simulink model "VehCtrl20260630_18B"  (R2018b)
settings: Solver=FixedStepAuto  StartTime=0.0  StopTime=inf  FixedStep=0.005  RelTol=1e-3
InitFcn:
  | mbd_mpc_consistency_checks(bdroot(gcs));
undefined symbols (not defined in the file): ANG_DEAD, BMS_NormalPwr, BrakeDeadZone, BrkPrsByBrkPct_TB_X, BrkPrsByBrkPct_TB_Y, DELAY_DISCHARGE, DELAY_RCUOFF, DRV_BACKWARD, DRV_BRAKE, DRV_FORWARD, DRV_NEUTRAL, DRV_PARK, DRV_UNPARK, DRV_ZEROTURN, EPB_LOCK, EPB_UNLOCK, ExtraLoadPwr, FanOff, fifo_0_vect, fifo_1_vect, HiFanReq, HV_finished, HV_No_Active, HV_POWER_OFF, HV_POWER_ON, HVDown, HVON, KaTLS_v_DrgUp_X_VehSpd, KeFTM_s_Way1OffDlyTime, KeFTM_TK_Way1CoolLv2OffBatTemp, KeFTM_TK_Way1CoolLv2OffMtrTemp, KeFTM_TK_Way1CoolLv2OnBatTemp, KeFTM_TK_Way1CoolLv2OnMtrTemp, KeFTM_TK_Way1CoolLv3OffBatTemp, KeFTM_TK_Way1CoolLv3OffMtrTemp, KeFTM_TK_Way1CoolLv3OnBatTemp, KeFTM_TK_Way1CoolLv3OnMtrTemp, KeFTM_TK_Way1CoolLv4OffBatTemp, KeFTM_TK_Way1CoolLv4OffMtrTemp, KeFTM_TK_Way1CoolLv4OnBatTemp, KeFTM_TK_Way1CoolLv4OnMtrTemp, Kp1, Kp2, LowFanReq, LQFP, MtrCmdGainFL, MtrCmdGainFR, MtrCmdGainRL, MtrCmdGainRR, MtrPwrFactor_RCU, MtrPwrHighToMidThd, MtrPwrLowToMidThd, MtrPwrMidToHighThd, MtrPwrMidToLowThd, MtrTrqMax, PCT_DEAD, Precharge, PTO_1000, PTO_540, pts1_fifo_0_vect ... (+32)
libraries: mbd_mpc574x_ec_toolbox x175, simulink x110, canmsglib x70
(part 2 of 15)

== system VehCtrl20260630_18B/Init ==
  CAN_init : Subsystem
  Data Store Read1 : DataStoreRead  DataStoreName=VCU_Mode
  Data Store Read3 : DataStoreRead  DataStoreName=Init_flg
  If1 : If  IfExpression=u1 == 2  ShowElse=off
  If2 : If  IfExpression=u1 == 0  ShowElse=off
  Init : Subsystem
  wires:
  Data Store Read3/1 -> If2/1
  If2/1 -> Init/Action
  Data Store Read1/1 -> If1/1
  If1/1 -> CAN_init/Action

== system VehCtrl20260630_18B/Initialization & SPI timer1 ==
  note: 由于SPI0用了两个片选，SPI3只用了一个片选（没算EEPROM）。
      | 因此直接用方波就可以了。
      | 如果增加SPI控制，建议使用StateFlow构造激活函数。
      | 由于模版使用的0.01s的仿真步长，这里构造周期为0.02s,占空比为0.5的方波。
  note: SPI3
  note: SPI0
  CS1 LS : Subsystem
  CS2 CANB : Subsystem
  CS3 LS : Subsystem
  CS5 LS : Subsystem
  Chart : Stateflow chart  TreatAsAtomicUnit=on
  Chart1 : Stateflow chart  TreatAsAtomicUnit=on
  Chart2 : Stateflow chart  TreatAsAtomicUnit=on
  Compare To Constant : simulink/Logic and Bit Operations/Compare To Constant  relop===  const=9  OutDataTypeStr=boolean
  Compare To Constant1 : simulink/Logic and Bit Operations/Compare To Constant  relop===  const=9  OutDataTypeStr=boolean
  Constant : Constant
  Data Store Read : DataStoreRead  DataStoreName=VCU_Mode
  Data Store Read1 : DataStoreRead  DataStoreName=ResetFlg
  Data Store Read2 : DataStoreRead  DataStoreName=Init_flg_SPI
  Data Store Write : DataStoreWrite  DataStoreName=VCU_Mode
  Data Store Write2 : DataStoreWrite  DataStoreName=SPI0_CS
  Data Store Write3 : DataStoreWrite  DataStoreName=SPI3_CS
  Data Store Write4 : DataStoreWrite  DataStoreName=Init_flg_SPI
  Data Type Conversion{,1..3} (4 alike) : DataTypeConversion
  If : If  IfExpression=u1 == 1  ShowElse=off
  If1 : If  IfExpression=u1 == 1  ShowElse=off
  If2 : If  IfExpression=u1 == 2  ShowElse=off
  If3 : If  IfExpression=u1 == 2  ShowElse=off
  Logical Operator : Logic  AllPortsSameDT=off  OutDataTypeStr=boolean
  Pulse Generator : DiscretePulseGenerator  PulseType=Time based  Period=0.01  PulseWidth=50
  wires:
  If/1 -> CS2 CANB/Action
  Chart/1(Flg) -> Data Type Conversion3/1
  Data Store Read2/1 -> Chart/2(InitFlg)
  If1/1 -> CS1 LS/Action
  Chart2/1(Flg) -> If3/1, [SPI3_flg], If/1
  Data Store Read/1 -> Chart2/1(VcuMode), Chart1/1(VcuMode)
  If2/1 -> CS5 LS/Action
  [SPI0_flg] -> Compare To Constant/1
  [SPI3_flg] -> Compare To Constant1/1
  Compare To Constant/1 -> Logical Operator/1
  Compare To Constant1/1 -> Logical Operator/2
  Logical Operator/1 -> Data Type Conversion2/1
  If3/1 -> CS3 LS/Action
  Pulse Generator/1 -> Data Type Conversion/1
  Constant/1 -> Data Type Conversion1/1
  Data Type Conversion/1 -> Data Store Write2/1
  Data Type Conversion1/1 -> Data Store Write3/1
  Data Type Conversion2/1 -> Data Store Write4/1
  Data Type Conversion3/1 -> Data Store Write/1
  Chart1/1(Flg) -> If1/1, [SPI0_flg], If2/1
  Data Store Read1/1 -> Chart/1(ResetFlg)

== system VehCtrl20260630_18B/Power Managment ==
  PowerMode : Inport
  Data Type Conversion : DataTypeConversion
  HS1 : mbd_mpc574x_ec_toolbox/GPIO Blocks/Digital_Output  Priority=1  gpio_pin=PTF6: [SIUL2_GPIO86 | General Purpose IO PF[6]]  gpio_drive_strength=Disabled
  HS4 : mbd_mpc574x_ec_toolbox/GPIO Blocks/Digital_Output  Priority=1  gpio_pin=PTA13: [SIUL2_GPIO13 | General Purpose IO PA[13]]  gpio_drive_strength=Disabled
  wires:
  PowerMode/1 -> Data Type Conversion/1
  Data Type Conversion/1 -> HS4/1, HS1/1

== system VehCtrl20260630_18B/SPI_EEPROM ==
  Data Store Memory : DataStoreMemory  DataStoreName=A_write  ReadBeforeWriteMsg=warning  WriteAfterWriteMsg=warning  WriteAfterReadMsg=warning  ShowAdditionalParam=off  OutDataTypeStr=single
      settings: RTWStateStorageClass=ExportedGlobal
  Data Store Memory10 : DataStoreMemory  DataStoreName=A_read  ReadBeforeWriteMsg=warning  WriteAfterWriteMsg=warning  WriteAfterReadMsg=warning  ShowAdditionalParam=off  OutDataTypeStr=single
      settings: RTWStateStorageClass=ExportedGlobal
  Data Store Memory18 : DataStoreMemory  DataStoreName=SPI0_CTRL0  ReadBeforeWriteMsg=warning  WriteAfterWriteMsg=warning  WriteAfterReadMsg=warning  ShowAdditionalParam=off  OutDataTypeStr=uint8
      settings: RTWStateStorageClass=ExportedGlobal
  Data Store Read : DataStoreRead  DataStoreName=SPI0_CTRL0
  SPI_read : Subsystem  TreatAsAtomicUnit=on
  SPI_write : Subsystem  TreatAsAtomicUnit=on
  Switch Case : SwitchCase  CaseConditions={1,2}  ShowDefaultCase=off
  wires:
  Data Store Read/1 -> Switch Case/1
  Switch Case/2 -> SPI_write/Action
  Switch Case/1 -> SPI_read/Action

== system VehCtrl20260630_18B/SigIn ==
  note: HardWareSignalIn
  note: CAN
  AI : Subsystem
  CAN0 : Subsystem  TreatAsAtomicUnit=on
      settings: RTWSystemCode=Nonreusable function
  CAN0_Rx_500 : mbd_mpc574x_ec_toolbox/Communication Blocks/CAN Blocks/FCAN_Isr  can_instance=0  can_event=Rx Complete
      settings: SourceProductName=NXP Model-Based Design Toolbox for MPC57xx MCUs
  CAN1 : Subsystem  TreatAsAtomicUnit=on
      settings: RTWSystemCode=Nonreusable function
  CAN1_Rx_500 : mbd_mpc574x_ec_toolbox/Communication Blocks/CAN Blocks/FCAN_Isr  can_instance=1  can_event=Rx Complete
      settings: SourceProductName=NXP Model-Based Design Toolbox for MPC57xx MCUs
  DI : Subsystem
  PWM : Subsystem
  Terminator{,3..5,8} (5 alike) : Terminator
  MCU_FL : Outport  VectorParamsAs1DForOutWhenUnconnected=on
  MCU_FR : Outport  Port=2  VectorParamsAs1DForOutWhenUnconnected=on
  MCU_RL : Outport  Port=3  VectorParamsAs1DForOutWhenUnconnected=on
  MCU_RR : Outport  Port=4  VectorParamsAs1DForOutWhenUnconnected=on
  MCU_PTO : Outport  Port=5  VectorParamsAs1DForOutWhenUnconnected=on
  BMS : Outport  Port=6  VectorParamsAs1DForOutWhenUnconnected=on
  DCDC : Outport  Port=7  VectorParamsAs1DForOutWhenUnconnected=on
  BDX : Outport  Port=8  VectorParamsAs1DForOutWhenUnconnected=on
  ACM : Outport  Port=9  VectorParamsAs1DForOutWhenUnconnected=on
  RCU : Outport  Port=10  VectorParamsAs1DForOutWhenUnconnected=on
  RMT : Outport  Port=11  VectorParamsAs1DForOutWhenUnconnected=on
  PTC : Outport  Port=12
  AUTO : Outport  Port=13  VectorParamsAs1DForOutWhenUnconnected=on
  wires:
  CAN0_Rx_500/2 -> Terminator4/1
  CAN0_Rx_500/6 -> CAN0/4(timestamp)
  CAN0_Rx_500/4 -> CAN0/2(Data)
  CAN0_Rx_500/3 -> CAN0/1(ID)
  CAN0_Rx_500/5 -> CAN0/3(length)
  CAN1_Rx_500/5 -> CAN1/3(length)
  CAN1_Rx_500/3 -> CAN1/1(ID)
  CAN1_Rx_500/4 -> CAN1/2(Data)
  CAN1_Rx_500/6 -> CAN1/4(timestamp)
  CAN1_Rx_500/1 -> CAN1/Trigger
  CAN1_Rx_500/2 -> Terminator8/1
  CAN1/1(MCU_FL) -> MCU_FL/1
  CAN1/2(MCU_FR) -> MCU_FR/1
  CAN1/4(MCU_RR) -> MCU_RR/1
  CAN1/3(MCU_RL) -> MCU_RL/1
  CAN0_Rx_500/1 -> CAN0/Trigger
  CAN1/5(MCU_PTO) -> MCU_PTO/1
  CAN1/6(BMS) -> BMS/1
  CAN1/7(BDX) -> BDX/1
  CAN0/3(DCDC) -> DCDC/1
  CAN1/8(ACM) -> ACM/1
  CAN1/9(RCU) -> RCU/1
  CAN0/1(PTC) -> PTC/1
  CAN0/4(RMT) -> RMT/1
  PWM/1(PWMIn) -> Terminator/1
  DI/1(DI) -> Terminator3/1
  AI/1(AI) -> Terminator5/1
  CAN0/2(AUTO) -> AUTO/1

== system VehCtrl20260630_18B/SigOut ==
  BMS_OUT : Inport
  RCU_OUT : Inport  Port=2
  DCDC_OUT : Inport  Port=3
  MCU_OUT : Inport  Port=4
  BDX_OUT : Inport  Port=5
  CAN_INFO : Inport  Port=6
  AUTO : Subsystem
  BDX : Subsystem  TreatAsAtomicUnit=on  SystemSampleTime=0.01
  BMS : Subsystem  TreatAsAtomicUnit=on  SystemSampleTime=0.01
  DCDC : Subsystem  TreatAsAtomicUnit=on  SystemSampleTime=0.01
  "GPIO " : Subsystem
  MCU : Subsystem  TreatAsAtomicUnit=on  SystemSampleTime=0.01
  METER : Subsystem
  PTC_ACM : Subsystem  TreatAsAtomicUnit=on  SystemSampleTime=0.01
  Pulse Generator : DiscretePulseGenerator  PulseType=Time based  Period=0.1  PulseWidth=5
  Pulse Generator1 : DiscretePulseGenerator  PulseType=Time based  Period=0.01  PulseWidth=50
  Pulse Generator2 : DiscretePulseGenerator  PulseType=Time based  Period=0.02  PulseWidth=25
  Pulse Generator3 : DiscretePulseGenerator  PulseType=Time based  Period=0.1  PulseWidth=5
  Pulse Generator4 : DiscretePulseGenerator  PulseType=Time based  Period=0.01  PulseWidth=50
  Pulse Generator5 : DiscretePulseGenerator  PulseType=Time based  Period=0.2  PulseWidth=50
  RCU : Subsystem  TreatAsAtomicUnit=on  SystemSampleTime=0.01
  Rate Transition{,1..5} (6 alike) : RateTransition
  wires:
  Rate Transition5/1 -> METER/1("CAN_INFO "), AUTO/1("CAN_INFO ")
  Pulse Generator2/1 -> BDX/Trigger
  Pulse Generator5/1 -> METER/Trigger
  BMS_OUT/1 -> Rate Transition/1
  Pulse Generator1/1 -> MCU/Trigger, RCU/Trigger
  MCU_OUT/1 -> Rate Transition3/1
  Pulse Generator3/1 -> PTC_ACM/Trigger
  Rate Transition2/1 -> DCDC/1("DCDC_OUT ")
  Rate Transition/1 -> BMS/1("BMS_OUT ")
  Rate Transition4/1 -> BDX/1("BDX_OUT ")
  RCU_OUT/1 -> Rate Transition1/1
  CAN_INFO/1 -> Rate Transition5/1
  Pulse Generator4/1 -> AUTO/Trigger
  Rate Transition1/1 -> RCU/1("RCU_OUT ")
  DCDC_OUT/1 -> Rate Transition2/1
  Pulse Generator/1 -> DCDC/Trigger, BMS/Trigger
  BDX_OUT/1 -> Rate Transition4/1
  Rate Transition3/1 -> MCU/1("MCU_OUT_FL ")

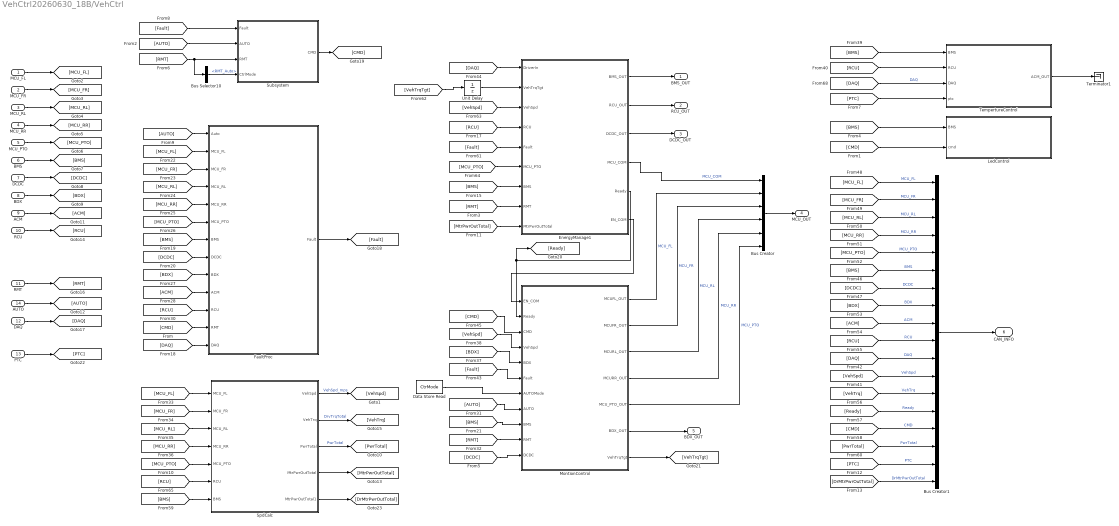
== system VehCtrl20260630_18B/VehCtrl ==
  MCU_FL : Inport
  MCU_FR : Inport  Port=2
  MCU_RL : Inport  Port=3
  MCU_RR : Inport  Port=4
  MCU_PTO : Inport  Port=5
  BMS : Inport  Port=6
  DCDC : Inport  Port=7
  BDX : Inport  Port=8
  ACM : Inport  Port=9
  RCU : Inport  Port=10
  RMT : Inport  Port=11
  DAQ : Inport  Port=12
  "PTC " : Inport  Port=13
  AUTO : Inport  Port=14
  Bus Creator : BusCreator  Inputs=6
  Bus Creator1 : BusCreator  Inputs=18
  Bus Selector10 : BusSelector  OutputSignals=RMT3.RMT_Auto
  Data Store Read : DataStoreRead  DataStoreName=CtrMode
  EnergyManage1 : Subsystem
  FaultProc : Subsystem
  LedControl : Subsystem
  MontionControl : Subsystem
  SpdCalc : Subsystem
  Subsystem : Subsystem
  TempertureControl : Subsystem
  Terminator1 : Terminator
  Unit Delay : UnitDelay  SampleTime=-1
  BMS_OUT : Outport
  RCU_OUT : Outport  Port=2
  DCDC_OUT : Outport  Port=3
  MCU_OUT : Outport  Port=4
  BDX_OUT : Outport  Port=5
  CAN_INFO : Outport  Port=6
  wires:
  MCU_FL/1 -> [MCU_FL]
  MCU_FR/1 -> [MCU_FR]
  MCU_RR/1 -> [MCU_RR]
  MCU_RL/1 -> [MCU_RL]
  DCDC/1 -> [DCDC]
  BDX/1 -> [BDX]
  BMS/1 -> [BMS]
  MCU_PTO/1 -> [MCU_PTO]
  RMT/1 -> [RMT]
  DAQ/1 -> [DAQ]
  RCU/1 -> [RCU]
  ACM/1 -> [ACM]
  [RCU] -> EnergyManage1/4(RCU)
  [MCU_FL] -> FaultProc/2(MCU_FL)
  [MCU_FR] -> FaultProc/3(MCU_FR)
  [MCU_RL] -> FaultProc/4(MCU_RL)
  [MCU_RR] -> FaultProc/5(MCU_RR)
  [MCU_PTO] -> FaultProc/6(MCU_PTO)
  [BMS] -> FaultProc/7(BMS)
  [DCDC] -> FaultProc/8(DCDC)
  [BDX] -> FaultProc/9(BDX)
  [ACM] -> FaultProc/10(ACM)
  [RCU] -> FaultProc/11(RCU)
  [CMD] -> FaultProc/12(RMT)
  [DAQ] -> FaultProc/13(DAQ)
  [BDX] -> MontionControl/5(BDX)
  [VehSpd] -> MontionControl/4(VehSpd)
  FaultProc/1(Fault) -> [Fault]
  [Fault] -> MontionControl/6(Fault)
  [DAQ] -> EnergyManage1/1(DriverIn)
  [CMD] -> MontionControl/3(CMD)
  [Fault] -> EnergyManage1/5(Fault)
  MontionControl/7(VehTrqTgt) -> [VehTrqTgt]
  [VehTrqTgt] -> Unit Delay/1
  [VehSpd] -> EnergyManage1/3(VehSpd)
  [MCU_PTO] -> EnergyManage1/6(MCU_PTO)
  [BMS] -> EnergyManage1/7(BMS)
  Unit Delay/1 -> EnergyManage1/2(VehTrqTgt)
  EnergyManage1/4(MCU_COM) -> Bus Creator/1  "MCU_COM"
  Bus Creator/1 -> MCU_OUT/1
  EnergyManage1/1(BMS_OUT) -> BMS_OUT/1
  EnergyManage1/2(RCU_OUT) -> RCU_OUT/1
  EnergyManage1/3(DCDC_OUT) -> DCDC_OUT/1
  MontionControl/1(MCUFL_OUT) -> Bus Creator/2  "MCU_FL"
  MontionControl/2(MCUFR_OUT) -> Bus Creator/3  "MCU_FR"
  MontionControl/3(MCURL_OUT) -> Bus Creator/4  "MCU_RL"
  MontionControl/4(MCURR_OUT) -> Bus Creator/5  "MCU_RR"
  MontionControl/5(MCU_PTO_OUT) -> Bus Creator/6  "MCU_PTO"
  MontionControl/6(BDX_OUT) -> BDX_OUT/1
  "PTC "/1 -> [PTC]
  AUTO/1 -> [AUTO]
  [AUTO] -> Subsystem/2(AUTO)
  Subsystem/1(CMD) -> [CMD]
  Data Store Read/1 -> MontionControl/7(AUTOMode)
  [AUTO] -> MontionControl/8(AUTO)
  Bus Selector10/1 -> Subsystem/4(CtrlMode)  "<RMT_Auto>"
  [RMT] -> Subsystem/3(RMT), Bus Selector10/1
  [RMT] -> EnergyManage1/8("RMT ")
  [CMD] -> LedControl/2(cmd)
  TempertureControl/1(ACM_OUT) -> Terminator1/1
  [RCU] -> TempertureControl/2(RCU)
  [BMS] -> TempertureControl/1(BMS)
  [BMS] -> MontionControl/9(BMS)
  [RMT] -> MontionControl/10(RMT)
  [DAQ] -> TempertureControl/3(DAQ)  "DAQ"
  [BMS] -> LedControl/1(BMS)
  [DCDC] -> MontionControl/11(DCDC)
  [PTC] -> TempertureControl/4(ptc)
  [Fault] -> Subsystem/1(Fault)
  [AUTO] -> FaultProc/1(Auto)
  [MCU_RR] -> SpdCalc/4(MCU_RR)
  [MCU_FR] -> SpdCalc/2(MCU_FR)
  [MCU_FL] -> SpdCalc/1(MCU_FL)
  [MCU_PTO] -> SpdCalc/5(MCU_PTO)
  [BMS] -> SpdCalc/7(BMS)
  SpdCalc/2("VehTrq ") -> [VehTrq]  "DrvTrqTotal"
  [RCU] -> SpdCalc/6(RCU)
  SpdCalc/5(MtrPwrOutTotal1) -> [DrMtrPwrOutTotal]
  SpdCalc/4(MtrPwrOutTotal) -> [MtrPwrOutTotal]
  SpdCalc/1(VehSpd) -> [VehSpd]  "VehSpd_mps"
  SpdCalc/3(PwrTotal) -> [PwrTotal]  "PwrTotal"
  [MCU_RL] -> SpdCalc/3(MCU_RL)
  EnergyManage1/6(EN_COM) -> MontionControl/1(EN_COM)
  EnergyManage1/5(Ready) -> MontionControl/2(Ready), [Ready]
  [MtrPwrOutTotal] -> EnergyManage1/9(MtrPwrOutTotal)
  Bus Creator1/1 -> CAN_INFO/1
  [BMS] -> Bus Creator1/6  "BMS"
  [MCU_FR] -> Bus Creator1/2  "MCU_FR"
  [PwrTotal] -> Bus Creator1/16  "PwrTotal"
  [MCU_RL] -> Bus Creator1/3  "MCU_RL"
  [DAQ] -> Bus Creator1/11  "DAQ"
  [BDX] -> Bus Creator1/8  "BDX"
  [MCU_RR] -> Bus Creator1/4  "MCU_RR"
  [VehSpd] -> Bus Creator1/12  "VehSpd"
  [CMD] -> Bus Creator1/15  "CMD"
  [DrMtrPwrOutTotal] -> Bus Creator1/18  "DrMtrPwrOutTotal"
  [ACM] -> Bus Creator1/9  "ACM"
  [Ready] -> Bus Creator1/14  "Ready"
  [MCU_PTO] -> Bus Creator1/5  "MCU_PTO"
  [PTC] -> Bus Creator1/17  "PTC"
  [DCDC] -> Bus Creator1/7  "DCDC"
  [MCU_FL] -> Bus Creator1/1  "MCU_FL"
  [VehTrq] -> Bus Creator1/13  "VehTrq"
  [RCU] -> Bus Creator1/10  "RCU"

== system VehCtrl20260630_18B/Init/CAN_init ==
  note: CAN1
  note: CAN2
  Action Port : ActionPort  ActionType=then
  ACM : mbd_mpc574x_ec_toolbox/Communication Blocks/CAN Blocks/FCAN_Receive  can_instance=2  can_mode=Non-blocking  can_timeout_ms=0  can_mb_idx=28  can_extended_id=off  can_is_remote=off  can_id=284  can_msg_mask=FFFFFFFF  show_adv_opts=off  can_use_rxfifo=off  can_fd_enable=off
      settings: SourceProductName=NXP Model-Based Design Toolbox for MPC57xx MCUs
  AUTO1 : mbd_mpc574x_ec_toolbox/Communication Blocks/CAN Blocks/FCAN_Receive  can_instance=1  can_mode=Non-blocking  can_timeout_ms=0  can_mb_idx=37  can_extended_id=on  can_is_remote=off  can_id=1001  can_msg_mask=FFFFFFFF  show_adv_opts=off  can_use_rxfifo=off  can_fd_enable=off
      settings: SourceProductName=NXP Model-Based Design Toolbox for MPC57xx MCUs
  AUTO2 : mbd_mpc574x_ec_toolbox/Communication Blocks/CAN Blocks/FCAN_Receive  can_instance=1  can_mode=Non-blocking  can_timeout_ms=0  can_mb_idx=38  can_extended_id=on  can_is_remote=off  can_id=1002  can_msg_mask=FFFFFFFF  show_adv_opts=off  can_use_rxfifo=off  can_fd_enable=off
      settings: SourceProductName=NXP Model-Based Design Toolbox for MPC57xx MCUs
  AUTO3 : mbd_mpc574x_ec_toolbox/Communication Blocks/CAN Blocks/FCAN_Receive  can_instance=1  can_mode=Non-blocking  can_timeout_ms=0  can_mb_idx=61  can_extended_id=on  can_is_remote=off  can_id=1003  can_msg_mask=FFFFFFFF  show_adv_opts=off  can_use_rxfifo=off  can_fd_enable=off
      settings: SourceProductName=NXP Model-Based Design Toolbox for MPC57xx MCUs
  "BDX " : mbd_mpc574x_ec_toolbox/Communication Blocks/CAN Blocks/FCAN_Receive  can_instance=2  can_mode=Non-blocking  can_timeout_ms=0  can_mb_idx=27  can_extended_id=off  can_is_remote=off  can_id=180  can_msg_mask=FFFFFFFF  show_adv_opts=off  can_use_rxfifo=off  can_fd_enable=off
      settings: SourceProductName=NXP Model-Based Design Toolbox for MPC57xx MCUs
  BMS1 : mbd_mpc574x_ec_toolbox/Communication Blocks/CAN Blocks/FCAN_Receive  can_instance=2  can_mode=Non-blocking  can_timeout_ms=0  can_mb_idx=20  can_extended_id=on  can_is_remote=off  can_id=18012947  can_msg_mask=FFFFFFFF  show_adv_opts=off  can_use_rxfifo=off  can_fd_enable=off
      settings: SourceProductName=NXP Model-Based Design Toolbox for MPC57xx MCUs
  BMS10 : mbd_mpc574x_ec_toolbox/Communication Blocks/CAN Blocks/FCAN_Receive  can_instance=2  can_mode=Non-blocking  can_timeout_ms=0  can_mb_idx=54  can_extended_id=on  can_is_remote=off  can_id=18022947  can_msg_mask=FFFFFFFF  show_adv_opts=off  can_use_rxfifo=off  can_fd_enable=off
      settings: SourceProductName=NXP Model-Based Design Toolbox for MPC57xx MCUs
  BMS11 : mbd_mpc574x_ec_toolbox/Communication Blocks/CAN Blocks/FCAN_Receive  can_instance=2  can_mode=Non-blocking  can_timeout_ms=0  can_mb_idx=55  can_extended_id=on  can_is_remote=off  can_id=18032947  can_msg_mask=FFFFFFFF  show_adv_opts=off  can_use_rxfifo=off  can_fd_enable=off
      settings: SourceProductName=NXP Model-Based Design Toolbox for MPC57xx MCUs
  BMS12 : mbd_mpc574x_ec_toolbox/Communication Blocks/CAN Blocks/FCAN_Receive  Commented=on  can_instance=2  can_mode=Non-blocking  can_timeout_ms=0  can_mb_idx=56  can_extended_id=on  can_is_remote=off  can_id=1C1F7547  can_msg_mask=FFFFFFFF  show_adv_opts=off  can_use_rxfifo=off  can_fd_enable=off
      settings: SourceProductName=NXP Model-Based Design Toolbox for MPC57xx MCUs
  BMS2 : mbd_mpc574x_ec_toolbox/Communication Blocks/CAN Blocks/FCAN_Receive  can_instance=2  can_mode=Non-blocking  can_timeout_ms=0  can_mb_idx=21  can_extended_id=on  can_is_remote=off  can_id=18042947  can_msg_mask=FFFFFFFF  show_adv_opts=off  can_use_rxfifo=off  can_fd_enable=off
      settings: SourceProductName=NXP Model-Based Design Toolbox for MPC57xx MCUs
  BMS3 : mbd_mpc574x_ec_toolbox/Communication Blocks/CAN Blocks/FCAN_Receive  can_instance=2  can_mode=Non-blocking  can_timeout_ms=0  can_mb_idx=22  can_extended_id=on  can_is_remote=off  can_id=18052947  can_msg_mask=FFFFFFFF  show_adv_opts=off  can_use_rxfifo=off  can_fd_enable=off
      settings: SourceProductName=NXP Model-Based Design Toolbox for MPC57xx MCUs
  BMS4 : mbd_mpc574x_ec_toolbox/Communication Blocks/CAN Blocks/FCAN_Receive  Commented=on  can_instance=2  can_mode=Non-blocking  can_timeout_ms=0  can_mb_idx=23  can_extended_id=on  can_is_remote=off  can_id=18062947  can_msg_mask=FFFFFFFF  show_adv_opts=off  can_use_rxfifo=off  can_fd_enable=off
      settings: SourceProductName=NXP Model-Based Design Toolbox for MPC57xx MCUs
  BMS5 : mbd_mpc574x_ec_toolbox/Communication Blocks/CAN Blocks/FCAN_Receive  can_instance=2  can_mode=Non-blocking  can_timeout_ms=0  can_mb_idx=24  can_extended_id=on  can_is_remote=off  can_id=1C017547  can_msg_mask=FFFFFFFF  show_adv_opts=off  can_use_rxfifo=off  can_fd_enable=off
      settings: SourceProductName=NXP Model-Based Design Toolbox for MPC57xx MCUs
  BMS6 : mbd_mpc574x_ec_toolbox/Communication Blocks/CAN Blocks/FCAN_Receive  can_instance=2  can_mode=Non-blocking  can_timeout_ms=0  can_mb_idx=50  can_extended_id=on  can_is_remote=off  can_id=1C067547  can_msg_mask=FFFFFFFF  show_adv_opts=off  can_use_rxfifo=off  can_fd_enable=off
      settings: SourceProductName=NXP Model-Based Design Toolbox for MPC57xx MCUs
  BMS7 : mbd_mpc574x_ec_toolbox/Communication Blocks/CAN Blocks/FCAN_Receive  Commented=on  can_instance=2  can_mode=Non-blocking  can_timeout_ms=0  can_mb_idx=51  can_extended_id=on  can_is_remote=off  can_id=180D2947  can_msg_mask=FFFFFFFF  show_adv_opts=off  can_use_rxfifo=off  can_fd_enable=off
      settings: SourceProductName=NXP Model-Based Design Toolbox for MPC57xx MCUs
  BMS8 : mbd_mpc574x_ec_toolbox/Communication Blocks/CAN Blocks/FCAN_Receive  can_instance=2  can_mode=Non-blocking  can_timeout_ms=0  can_mb_idx=52  can_extended_id=on  can_is_remote=off  can_id=18602947  can_msg_mask=FFFFFFFF  show_adv_opts=off  can_use_rxfifo=off  can_fd_enable=off
      settings: SourceProductName=NXP Model-Based Design Toolbox for MPC57xx MCUs
  BMS9 : mbd_mpc574x_ec_toolbox/Communication Blocks/CAN Blocks/FCAN_Receive  can_instance=2  can_mode=Non-blocking  can_timeout_ms=0  can_mb_idx=53  can_extended_id=on  can_is_remote=off  can_id=18202947  can_msg_mask=FFFFFFFF  show_adv_opts=off  can_use_rxfifo=off  can_fd_enable=off
      settings: SourceProductName=NXP Model-Based Design Toolbox for MPC57xx MCUs
  DCDC : mbd_mpc574x_ec_toolbox/Communication Blocks/CAN Blocks/FCAN_Receive  can_instance=1  can_mode=Non-blocking  can_timeout_ms=0  can_mb_idx=26  can_extended_id=on  can_is_remote=off  can_id=18F8622B  can_msg_mask=FFFFFFFF  show_adv_opts=off  can_use_rxfifo=off  can_fd_enable=off
      settings: SourceProductName=NXP Model-Based Design Toolbox for MPC57xx MCUs
  MCU_FL1 : mbd_mpc574x_ec_toolbox/Communication Blocks/CAN Blocks/FCAN_Receive  can_instance=2  can_mode=Non-blocking  can_timeout_ms=0  can_mb_idx=12  can_extended_id=on  can_is_remote=off  can_id=C08A7F3  can_msg_mask=FFFFFFFF  show_adv_opts=off  can_use_rxfifo=off  can_fd_enable=off
      settings: SourceProductName=NXP Model-Based Design Toolbox for MPC57xx MCUs
  MCU_FL2 : mbd_mpc574x_ec_toolbox/Communication Blocks/CAN Blocks/FCAN_Receive  can_instance=2  can_mode=Non-blocking  can_timeout_ms=0  can_mb_idx=13  can_extended_id=on  can_is_remote=off  can_id=C09A7F3  can_msg_mask=FFFFFFFF  show_adv_opts=off  can_use_rxfifo=off  can_fd_enable=off
      settings: SourceProductName=NXP Model-Based Design Toolbox for MPC57xx MCUs
  MCU_FL3 : mbd_mpc574x_ec_toolbox/Communication Blocks/CAN Blocks/FCAN_Receive  can_instance=2  can_mode=Non-blocking  can_timeout_ms=0  can_mb_idx=14  can_extended_id=on  can_is_remote=off  can_id=C0AA7F3  can_msg_mask=FFFFFFFF  show_adv_opts=off  can_use_rxfifo=off  can_fd_enable=off
      settings: SourceProductName=NXP Model-Based Design Toolbox for MPC57xx MCUs
  MCU_FL4 : mbd_mpc574x_ec_toolbox/Communication Blocks/CAN Blocks/FCAN_Receive  Commented=on  can_instance=2  can_mode=Non-blocking  can_timeout_ms=0  can_mb_idx=15  can_extended_id=on  can_is_remote=off  can_id=C0BA7F3  can_msg_mask=FFFFFFFF  show_adv_opts=off  can_use_rxfifo=off  can_fd_enable=off
      settings: SourceProductName=NXP Model-Based Design Toolbox for MPC57xx MCUs
  MCU_FR1 : mbd_mpc574x_ec_toolbox/Communication Blocks/CAN Blocks/FCAN_Receive  can_instance=2  can_mode=Non-blocking  can_timeout_ms=0  can_mb_idx=0  can_extended_id=on  can_is_remote=off  can_id=C08A7F0  can_msg_mask=FFFFFFFF  show_adv_opts=off  can_use_rxfifo=off  can_fd_enable=off
      settings: SourceProductName=NXP Model-Based Design Toolbox for MPC57xx MCUs
  MCU_FR2 : mbd_mpc574x_ec_toolbox/Communication Blocks/CAN Blocks/FCAN_Receive  can_instance=2  can_mode=Non-blocking  can_timeout_ms=0  can_mb_idx=1  can_extended_id=on  can_is_remote=off  can_id=C09A7F0  can_msg_mask=FFFFFFFF  show_adv_opts=off  can_use_rxfifo=off  can_fd_enable=off
      settings: SourceProductName=NXP Model-Based Design Toolbox for MPC57xx MCUs
  MCU_FR3 : mbd_mpc574x_ec_toolbox/Communication Blocks/CAN Blocks/FCAN_Receive  can_instance=2  can_mode=Non-blocking  can_timeout_ms=0  can_mb_idx=2  can_extended_id=on  can_is_remote=off  can_id=C0AA7F0  can_msg_mask=FFFFFFFF  show_adv_opts=off  can_use_rxfifo=off  can_fd_enable=off
      settings: SourceProductName=NXP Model-Based Design Toolbox for MPC57xx MCUs
  MCU_FR4 : mbd_mpc574x_ec_toolbox/Communication Blocks/CAN Blocks/FCAN_Receive  Commented=on  can_instance=2  can_mode=Non-blocking  can_timeout_ms=0  can_mb_idx=3  can_extended_id=on  can_is_remote=off  can_id=C0BA7F0  can_msg_mask=FFFFFFFF  show_adv_opts=off  can_use_rxfifo=off  can_fd_enable=off
      settings: SourceProductName=NXP Model-Based Design Toolbox for MPC57xx MCUs
  MCU_PTO1 : mbd_mpc574x_ec_toolbox/Communication Blocks/CAN Blocks/FCAN_Receive  can_instance=2  can_mode=Non-blocking  can_timeout_ms=0  can_mb_idx=16  can_extended_id=on  can_is_remote=off  can_id=C08A7F4  can_msg_mask=FFFFFFFF  show_adv_opts=off  can_use_rxfifo=off  can_fd_enable=off
      settings: SourceProductName=NXP Model-Based Design Toolbox for MPC57xx MCUs
  MCU_PTO2 : mbd_mpc574x_ec_toolbox/Communication Blocks/CAN Blocks/FCAN_Receive  can_instance=2  can_mode=Non-blocking  can_timeout_ms=0  can_mb_idx=17  can_extended_id=on  can_is_remote=off  can_id=C09A7F4  can_msg_mask=FFFFFFFF  show_adv_opts=off  can_use_rxfifo=off  can_fd_enable=off
      settings: SourceProductName=NXP Model-Based Design Toolbox for MPC57xx MCUs
  MCU_PTO3 : mbd_mpc574x_ec_toolbox/Communication Blocks/CAN Blocks/FCAN_Receive  can_instance=2  can_mode=Non-blocking  can_timeout_ms=0  can_mb_idx=18  can_extended_id=on  can_is_remote=off  can_id=C0AA7F4  can_msg_mask=FFFFFFFF  show_adv_opts=off  can_use_rxfifo=off  can_fd_enable=off
      settings: SourceProductName=NXP Model-Based Design Toolbox for MPC57xx MCUs
  MCU_PTO4 : mbd_mpc574x_ec_toolbox/Communication Blocks/CAN Blocks/FCAN_Receive  Commented=on  can_instance=2  can_mode=Non-blocking  can_timeout_ms=0  can_mb_idx=19  can_extended_id=on  can_is_remote=off  can_id=C0BA7F4  can_msg_mask=FFFFFFFF  show_adv_opts=off  can_use_rxfifo=off  can_fd_enable=off
      settings: SourceProductName=NXP Model-Based Design Toolbox for MPC57xx MCUs
  MCU_RL1 : mbd_mpc574x_ec_toolbox/Communication Blocks/CAN Blocks/FCAN_Receive  can_instance=2  can_mode=Non-blocking  can_timeout_ms=0  can_mb_idx=8  can_extended_id=on  can_is_remote=off  can_id=C08A7F2  can_msg_mask=FFFFFFFF  show_adv_opts=off  can_use_rxfifo=off  can_fd_enable=off
      settings: SourceProductName=NXP Model-Based Design Toolbox for MPC57xx MCUs
  MCU_RL2 : mbd_mpc574x_ec_toolbox/Communication Blocks/CAN Blocks/FCAN_Receive  can_instance=2  can_mode=Non-blocking  can_timeout_ms=0  can_mb_idx=9  can_extended_id=on  can_is_remote=off  can_id=C09A7F2  can_msg_mask=FFFFFFFF  show_adv_opts=off  can_use_rxfifo=off  can_fd_enable=off
      settings: SourceProductName=NXP Model-Based Design Toolbox for MPC57xx MCUs
  MCU_RL3 : mbd_mpc574x_ec_toolbox/Communication Blocks/CAN Blocks/FCAN_Receive  can_instance=2  can_mode=Non-blocking  can_timeout_ms=0  can_mb_idx=10  can_extended_id=on  can_is_remote=off  can_id=C0AA7F2  can_msg_mask=FFFFFFFF  show_adv_opts=off  can_use_rxfifo=off  can_fd_enable=off
      settings: SourceProductName=NXP Model-Based Design Toolbox for MPC57xx MCUs
  MCU_RL4 : mbd_mpc574x_ec_toolbox/Communication Blocks/CAN Blocks/FCAN_Receive  Commented=on  can_instance=2  can_mode=Non-blocking  can_timeout_ms=0  can_mb_idx=11  can_extended_id=on  can_is_remote=off  can_id=C0BA7F2  can_msg_mask=FFFFFFFF  show_adv_opts=off  can_use_rxfifo=off  can_fd_enable=off
      settings: SourceProductName=NXP Model-Based Design Toolbox for MPC57xx MCUs
  MCU_RR1 : mbd_mpc574x_ec_toolbox/Communication Blocks/CAN Blocks/FCAN_Receive  can_instance=2  can_mode=Non-blocking  can_timeout_ms=0  can_mb_idx=4  can_extended_id=on  can_is_remote=off  can_id=C08A7F1  can_msg_mask=FFFFFFFF  show_adv_opts=off  can_use_rxfifo=off  can_fd_enable=off
      settings: SourceProductName=NXP Model-Based Design Toolbox for MPC57xx MCUs
  MCU_RR2 : mbd_mpc574x_ec_toolbox/Communication Blocks/CAN Blocks/FCAN_Receive  can_instance=2  can_mode=Non-blocking  can_timeout_ms=0  can_mb_idx=5  can_extended_id=on  can_is_remote=off  can_id=C09A7F1  can_msg_mask=FFFFFFFF  show_adv_opts=off  can_use_rxfifo=off  can_fd_enable=off
      settings: SourceProductName=NXP Model-Based Design Toolbox for MPC57xx MCUs
  MCU_RR3 : mbd_mpc574x_ec_toolbox/Communication Blocks/CAN Blocks/FCAN_Receive  can_instance=2  can_mode=Non-blocking  can_timeout_ms=0  can_mb_idx=6  can_extended_id=on  can_is_remote=off  can_id=C0AA7F1  can_msg_mask=FFFFFFFF  show_adv_opts=off  can_use_rxfifo=off  can_fd_enable=off
      settings: SourceProductName=NXP Model-Based Design Toolbox for MPC57xx MCUs
  MCU_RR4 : mbd_mpc574x_ec_toolbox/Communication Blocks/CAN Blocks/FCAN_Receive  Commented=on  can_instance=2  can_mode=Non-blocking  can_timeout_ms=0  can_mb_idx=7  can_extended_id=on  can_is_remote=off  can_id=C0BA7F1  can_msg_mask=FFFFFFFF  show_adv_opts=off  can_use_rxfifo=off  can_fd_enable=off
      settings: SourceProductName=NXP Model-Based Design Toolbox for MPC57xx MCUs
  PTC1 : mbd_mpc574x_ec_toolbox/Communication Blocks/CAN Blocks/FCAN_Receive  can_instance=1  can_mode=Non-blocking  can_timeout_ms=0  can_mb_idx=23  can_extended_id=off  can_is_remote=off  can_id=49B  can_msg_mask=FFFFFFFF  show_adv_opts=off  can_use_rxfifo=off  can_fd_enable=off
      settings: SourceProductName=NXP Model-Based Design Toolbox for MPC57xx MCUs
  PTC2 : mbd_mpc574x_ec_toolbox/Communication Blocks/CAN Blocks/FCAN_Receive  Commented=on  can_instance=1  can_mode=Non-blocking  can_timeout_ms=0  can_mb_idx=47  can_extended_id=on  can_is_remote=off  can_id=49C  can_msg_mask=FFFFFFFF  show_adv_opts=off  can_use_rxfifo=off  can_fd_enable=off
      settings: SourceProductName=NXP Model-Based Design Toolbox for MPC57xx MCUs
  RCU1 : mbd_mpc574x_ec_toolbox/Communication Blocks/CAN Blocks/FCAN_Receive  can_instance=2  can_mode=Non-blocking  can_timeout_ms=0  can_mb_idx=29  can_extended_id=on  can_is_remote=off  can_id=18F0011B  can_msg_mask=FFFFFFFF  show_adv_opts=off  can_use_rxfifo=off  can_fd_enable=off
      settings: SourceProductName=NXP Model-Based Design Toolbox for MPC57xx MCUs
  RCU2 : mbd_mpc574x_ec_toolbox/Communication Blocks/CAN Blocks/FCAN_Receive  can_instance=2  can_mode=Non-blocking  can_timeout_ms=0  can_mb_idx=30  can_extended_id=on  can_is_remote=off  can_id=18F0022B  can_msg_mask=FFFFFFFF  show_adv_opts=off  can_use_rxfifo=off  can_fd_enable=off
      settings: SourceProductName=NXP Model-Based Design Toolbox for MPC57xx MCUs
  RCU3 : mbd_mpc574x_ec_toolbox/Communication Blocks/CAN Blocks/FCAN_Receive  can_instance=2  can_mode=Non-blocking  can_timeout_ms=0  can_mb_idx=31  can_extended_id=on  can_is_remote=off  can_id=18F0033B  can_msg_mask=FFFFFFFF  show_adv_opts=off  can_use_rxfifo=off  can_fd_enable=off
      settings: SourceProductName=NXP Model-Based Design Toolbox for MPC57xx MCUs
  RMT1 : mbd_mpc574x_ec_toolbox/Communication Blocks/CAN Blocks/FCAN_Receive  can_instance=1  can_mode=Non-blocking  can_timeout_ms=0  can_mb_idx=33  can_extended_id=off  can_is_remote=off  can_id=1  can_msg_mask=FFFFFFFF  show_adv_opts=off  can_use_rxfifo=off  can_fd_enable=off
      settings: SourceProductName=NXP Model-Based Design Toolbox for MPC57xx MCUs
  RMT2 : mbd_mpc574x_ec_toolbox/Communication Blocks/CAN Blocks/FCAN_Receive  can_instance=1  can_mode=Non-blocking  can_timeout_ms=0  can_mb_idx=34  can_extended_id=off  can_is_remote=off  can_id=2  can_msg_mask=FFFFFFFF  show_adv_opts=off  can_use_rxfifo=off  can_fd_enable=off
      settings: SourceProductName=NXP Model-Based Design Toolbox for MPC57xx MCUs
  RMT3 : mbd_mpc574x_ec_toolbox/Communication Blocks/CAN Blocks/FCAN_Receive  can_instance=1  can_mode=Non-blocking  can_timeout_ms=0  can_mb_idx=35  can_extended_id=off  can_is_remote=off  can_id=3  can_msg_mask=FFFFFFFF  show_adv_opts=off  can_use_rxfifo=off  can_fd_enable=off
      settings: SourceProductName=NXP Model-Based Design Toolbox for MPC57xx MCUs
  RMT4 : mbd_mpc574x_ec_toolbox/Communication Blocks/CAN Blocks/FCAN_Receive  can_instance=1  can_mode=Non-blocking  can_timeout_ms=0  can_mb_idx=36  can_extended_id=off  can_is_remote=off  can_id=4  can_msg_mask=FFFFFFFF  show_adv_opts=off  can_use_rxfifo=off  can_fd_enable=off
      settings: SourceProductName=NXP Model-Based Design Toolbox for MPC57xx MCUs
  RMT5 : mbd_mpc574x_ec_toolbox/Communication Blocks/CAN Blocks/FCAN_Receive  can_instance=1  can_mode=Non-blocking  can_timeout_ms=0  can_mb_idx=32  can_extended_id=off  can_is_remote=off  can_id=235  can_msg_mask=FFFFFFFF  show_adv_opts=off  can_use_rxfifo=off  can_fd_enable=off
      settings: SourceProductName=NXP Model-Based Design Toolbox for MPC57xx MCUs
  SENSOR : mbd_mpc574x_ec_toolbox/Communication Blocks/CAN Blocks/FCAN_Receive  can_instance=2  can_mode=Non-blocking  can_timeout_ms=0  can_mb_idx=25  can_extended_id=off  can_is_remote=off  can_id=585  can_msg_mask=FFFFFFFF  show_adv_opts=off  can_use_rxfifo=off  can_fd_enable=off
      settings: SourceProductName=NXP Model-Based Design Toolbox for MPC57xx MCUs

== system VehCtrl20260630_18B/Init/Init ==
  note: MainRelay
  Action Port : ActionPort  ActionType=then
  Constant : Constant
  Constant2 : Constant
  Data Store Write : DataStoreWrite  DataStoreName=LS001
  Data Store Write3 : DataStoreWrite  DataStoreName=Init_flg
  Data Type Conversion : DataTypeConversion
  Data Type Conversion2 : DataTypeConversion
  wires:
  Constant/1 -> Data Type Conversion/1
  Data Type Conversion/1 -> Data Store Write3/1
  Constant2/1 -> Data Type Conversion2/1
  Data Type Conversion2/1 -> Data Store Write/1

== system VehCtrl20260630_18B/Initialization & SPI timer1/CS1 LS ==
  Action Port : ActionPort  ActionType=then
  Chart : Stateflow chart  TreatAsAtomicUnit=on
  Data Type Conversion{,1,3..4} (4 alike) : DataTypeConversion
  Demux1 : Demux  Outputs=2
  SPI_Master_Transfer_To1 : mbd_mpc574x_ec_toolbox/Communication Blocks/SPI Blocks/SPI_Master_Transfer  Priority=2  InstanceNumber=0  xfermode=Non blocking  timeout=50  spi_upd=on  WhichPCS=5
  Subsystem : Subsystem  Commented=on
  Terminator : Terminator
  Terminator1 : Terminator
  Vector Concatenate1 : Concatenate
  wires:
  SPI_Master_Transfer_To1/1 -> Demux1/1
  Data Type Conversion3/1 -> Terminator/1
  Vector Concatenate1/1 -> SPI_Master_Transfer_To1/1
  Demux1/2 -> Data Type Conversion4/1
  Data Type Conversion4/1 -> Terminator1/1
  Demux1/1 -> Data Type Conversion3/1
  Chart/1(high) -> Data Type Conversion/1
  Chart/2(low) -> Data Type Conversion1/1
  Data Type Conversion/1 -> Vector Concatenate1/1
  Data Type Conversion1/1 -> Vector Concatenate1/2

== system VehCtrl20260630_18B/Initialization & SPI timer1/CS2 CANB ==
  Action Port : ActionPort  ActionType=then
  Constant : Constant  Value=2
  Constant1 : Constant  Value=7
  Data Type Conversion : DataTypeConversion  OutDataTypeStr=uint8
  Data Type Conversion1 : DataTypeConversion  OutDataTypeStr=uint8
  Data Type Conversion2 : DataTypeConversion
  Data Type Conversion3 : DataTypeConversion
  Demux2 : Demux  Outputs=2
  SPI_Master_Transfer_To2 : mbd_mpc574x_ec_toolbox/Communication Blocks/SPI Blocks/SPI_Master_Transfer  Priority=2  InstanceNumber=3  xfermode=Non blocking  timeout=50  spi_upd=on  WhichPCS=2
  Terminator : Terminator
  Terminator1 : Terminator
  Vector Concatenate2 : Concatenate
  wires:
  Vector Concatenate2/1 -> SPI_Master_Transfer_To2/1
  Demux2/2 -> Data Type Conversion1/1
  Data Type Conversion2/1 -> Vector Concatenate2/2
  SPI_Master_Transfer_To2/1 -> Demux2/1
  Data Type Conversion1/1 -> Terminator1/1
  Data Type Conversion/1 -> Terminator/1
  Demux2/1 -> Data Type Conversion/1
  Data Type Conversion3/1 -> Vector Concatenate2/1
  Constant/1 -> Data Type Conversion3/1
  Constant1/1 -> Data Type Conversion2/1

== system VehCtrl20260630_18B/Initialization & SPI timer1/CS3 LS ==
  note: 80-0101 0000 - 对A组端口控制模式进行设置
      | 96-0110 0000 - 对B组端口控制模式进行设置
      | 40-0010 1100 -使用SPI控制端口
      |
      | 其中端口1,2,5,6即为复用PWM端口，这里设置为引脚控制（A组），其余端口设置为SPI控制
  Action Port : ActionPort  ActionType=then
  Chart : Stateflow chart  TreatAsAtomicUnit=on
  Data Type Conversion : DataTypeConversion  OutDataTypeStr=uint8
  Data Type Conversion1 : DataTypeConversion  OutDataTypeStr=uint8
  Data Type Conversion2 : DataTypeConversion
  Data Type Conversion3 : DataTypeConversion
  Demux2 : Demux  Outputs=2
  Manual Switch : ManualSwitch  CurrentSetting=0
  PIN : Constant  Value=2
  SPI : Constant  Value=0
  SPI_Master_Transfer_To2 : mbd_mpc574x_ec_toolbox/Communication Blocks/SPI Blocks/SPI_Master_Transfer  Priority=2  InstanceNumber=3  xfermode=Non blocking  timeout=50  spi_upd=on  WhichPCS=3
  Subsystem : Subsystem  Commented=on
  Terminator2 : Terminator
  Terminator3 : Terminator
  Vector Concatenate1 : Concatenate
  wires:
  Data Type Conversion1/1 -> Terminator3/1
  Data Type Conversion/1 -> Terminator2/1
  Demux2/1 -> Data Type Conversion/1
  SPI_Master_Transfer_To2/1 -> Demux2/1
  Demux2/2 -> Data Type Conversion1/1
  Chart/2(low) -> Data Type Conversion3/1
  Vector Concatenate1/1 -> SPI_Master_Transfer_To2/1
  Data Type Conversion2/1 -> Vector Concatenate1/1
  Data Type Conversion3/1 -> Vector Concatenate1/2
  Chart/1(high) -> Data Type Conversion2/1
  PIN/1 -> Manual Switch/2
  SPI/1 -> Manual Switch/1
  Manual Switch/1 -> [Mode]
  [Mode] -> Chart/1(mode)

== system VehCtrl20260630_18B/Initialization & SPI timer1/CS5 LS ==
  Action Port : ActionPort  ActionType=then
  Chart : Stateflow chart  TreatAsAtomicUnit=on
  Data Type Conversion{,1,3..4} (4 alike) : DataTypeConversion
  Demux1 : Demux  Outputs=2
  SPI_Master_Transfer_To1 : mbd_mpc574x_ec_toolbox/Communication Blocks/SPI Blocks/SPI_Master_Transfer  Priority=2  InstanceNumber=0  xfermode=Non blocking  timeout=50  spi_upd=on  WhichPCS=1
  Subsystem : Subsystem  Commented=on
  Terminator : Terminator
  Terminator1 : Terminator
  Vector Concatenate1 : Concatenate
  wires:
  SPI_Master_Transfer_To1/1 -> Demux1/1
  Demux1/1 -> Data Type Conversion3/1
  Data Type Conversion3/1 -> Terminator/1
  Demux1/2 -> Data Type Conversion4/1
  Data Type Conversion4/1 -> Terminator1/1
  Chart/2(low) -> Data Type Conversion1/1
  Vector Concatenate1/1 -> SPI_Master_Transfer_To1/1
  Data Type Conversion/1 -> Vector Concatenate1/1
  Data Type Conversion1/1 -> Vector Concatenate1/2
  Chart/1(high) -> Data Type Conversion/1

== system VehCtrl20260630_18B/SPI_EEPROM/SPI_read ==
  Action Port : ActionPort
  "Address_High " : Constant  Value=hex2dec('FF')  OutDataTypeStr=uint8
  Address_Low : Constant  Value=hex2dec('FF')
  Bitwise AND : simulink/Logic and Bit Operations/Bitwise Operator  logicop=AND  UseBitMask=on  BitMask=hex2dec('00FF')  BitMaskRealWorld=Stored Integer
  Constant : Constant  Value=0
  Data Store Write : DataStoreWrite  DataStoreName=A_read
  Data Type Conversion{,1,3..8} (8 alike) : DataTypeConversion  OutDataTypeStr=uint8
  Data Type Conversion2 : DataTypeConversion
  Demux1 : Demux
  SPI_Master_Transfer_To1 : mbd_mpc574x_ec_toolbox/Communication Blocks/SPI Blocks/SPI_Master_Transfer  Priority=2  InstanceNumber=0  xfermode=Non blocking  timeout=50  spi_upd=on  WhichPCS=0
  Terminator : Terminator
  Terminator1 : Terminator
  Terminator2 : Terminator
  Vector Concatenate1 : Concatenate  NumInputs=4
  read_set : Constant  Value=3  OutDataTypeStr=uint8
  wires:
  "Address_High "/1 -> Data Type Conversion1/1
  read_set/1 -> Data Type Conversion/1
  Data Type Conversion1/1 -> Vector Concatenate1/2  "d1"
  Data Type Conversion/1 -> Vector Concatenate1/1  "d0"
  Address_Low/1 -> Data Type Conversion6/1
  Demux1/2 -> Data Type Conversion4/1
  Vector Concatenate1/1 -> SPI_Master_Transfer_To1/1
  Demux1/1 -> Data Type Conversion3/1
  SPI_Master_Transfer_To1/1 -> Demux1/1
  Data Type Conversion3/1 -> Terminator/1  "r0"
  Data Type Conversion8/1 -> Bitwise AND/1  "r3"
  Bitwise AND/1 -> Data Type Conversion2/1
  Data Type Conversion2/1 -> Data Store Write/1
  Constant/1 -> Data Type Conversion7/1
  Data Type Conversion6/1 -> Vector Concatenate1/3  "d2"
  Data Type Conversion7/1 -> Vector Concatenate1/4  "d3"
  Demux1/3 -> Data Type Conversion5/1
  Data Type Conversion4/1 -> Terminator1/1  "r1"
  Data Type Conversion5/1 -> Terminator2/1  "r2"
  Demux1/4 -> Data Type Conversion8/1

== system VehCtrl20260630_18B/SPI_EEPROM/SPI_write ==
  Action Port : ActionPort
  Data Store Memory : DataStoreMemory  DataStoreName=Write_Ctrl  ReadBeforeWriteMsg=warning  WriteAfterWriteMsg=warning  WriteAfterReadMsg=warning  InitialValue=1  ShowAdditionalParam=off  OutDataTypeStr=uint8
      settings: RTWStateStorageClass=ExportedGlobal
  Data Store Read : DataStoreRead  DataStoreName=Write_Ctrl
  SPI_enable : Subsystem  TreatAsAtomicUnit=on
  SPI_write : Subsystem  TreatAsAtomicUnit=on
  Switch Case : SwitchCase  CaseConditions={1,2}  ShowDefaultCase=off
  wires:
  Data Store Read/1 -> Switch Case/1
  Switch Case/2 -> SPI_write/Action
  Switch Case/1 -> SPI_enable/Action

== system VehCtrl20260630_18B/SigIn/AI ==
  note: 32V
  ADC_Start : mbd_mpc574x_ec_toolbox/Motor Control Blocks/ADC Blocks/ADC_Start  adc_instance=1  interrupt=off  presample=off
  ADC_Start1 : mbd_mpc574x_ec_toolbox/Motor Control Blocks/ADC Blocks/ADC_Start  adc_instance=0  interrupt=off  presample=off
  Bus Creator : BusCreator  Inputs=15
  Data Store Read : DataStoreRead  DataStoreName=AI18
  Data Store Read1 : DataStoreRead  DataStoreName=AI11
  Data Store Read10 : DataStoreRead  DataStoreName=AI17
  Data Store Read11 : DataStoreRead  DataStoreName=AI06
  Data Store Read12 : DataStoreRead  DataStoreName=AI12
  Data Store Read13 : DataStoreRead  DataStoreName=AI19
  Data Store Read14 : DataStoreRead  DataStoreName=AI07
  Data Store Read2 : DataStoreRead  DataStoreName=AI16
  Data Store Read3 : DataStoreRead  DataStoreName=AI20
  Data Store Read4 : DataStoreRead  DataStoreName=AI05
  Data Store Read5 : DataStoreRead  DataStoreName=AI03
  Data Store Read6 : DataStoreRead  DataStoreName=AI04
  Data Store Read7 : DataStoreRead  DataStoreName=AI09
  Data Store Read8 : DataStoreRead  DataStoreName=AI15
  Data Store Read9 : DataStoreRead  DataStoreName=AI08
  Data Store Write : DataStoreWrite  DataStoreName=AI11
  Data Store Write1 : DataStoreWrite  DataStoreName=AI16
  Data Store Write10 : DataStoreWrite  DataStoreName=AI03
  Data Store Write11 : DataStoreWrite  DataStoreName=AI04
  Data Store Write12 : DataStoreWrite  DataStoreName=AI05
  Data Store Write13 : DataStoreWrite  DataStoreName=AI09
  Data Store Write14 : DataStoreWrite  DataStoreName=AI20
  Data Store Write2 : DataStoreWrite  DataStoreName=AI18
  Data Store Write3 : DataStoreWrite  DataStoreName=AI06
  Data Store Write4 : DataStoreWrite  DataStoreName=AI07
  Data Store Write5 : DataStoreWrite  DataStoreName=AI08
  Data Store Write6 : DataStoreWrite  DataStoreName=AI12
  Data Store Write7 : DataStoreWrite  DataStoreName=AI15
  Data Store Write8 : DataStoreWrite  DataStoreName=AI17
  Data Store Write9 : DataStoreWrite  DataStoreName=AI19
  Data Type Conversion{,1..14} (15 alike) : DataTypeConversion  OutDataTypeStr=single
  Demux : Demux  Outputs=10
  Demux1 : Demux  Outputs=5
  Gain{1,6,8,10,12..14} (7 alike) : Gain  Gain=5/4095
  Gain{2..5,7,9,11,15} (8 alike) : Gain  Gain=36.6/4095  OutDataTypeStr=single
  AI : Outport
  wires:
  Demux/4 -> Data Type Conversion3/1
  ADC_Start1/1 -> Demux/1
  Demux/7 -> Data Type Conversion6/1
  Demux1/4 -> Data Type Conversion13/1
  Demux1/3 -> Data Type Conversion12/1
  ADC_Start/1 -> Demux1/1
  Demux1/2 -> Data Type Conversion11/1
  Demux1/5 -> Data Type Conversion14/1
  Demux1/1 -> Data Type Conversion10/1
  Demux/1 -> Data Type Conversion/1
  Demux/3 -> Data Type Conversion2/1
  Demux/2 -> Data Type Conversion1/1
  Demux/5 -> Data Type Conversion4/1
  Demux/8 -> Data Type Conversion7/1
  Demux/9 -> Data Type Conversion8/1
  Demux/10 -> Data Type Conversion9/1
  Demux/6 -> Data Type Conversion5/1
  Data Type Conversion/1 -> Gain6/1
  Gain6/1 -> Data Store Write7/1
  Data Type Conversion1/1 -> Gain7/1
  Data Type Conversion2/1 -> Gain1/1
  Data Type Conversion3/1 -> Gain2/1
  Data Type Conversion4/1 -> Gain8/1
  Data Type Conversion5/1 -> Gain3/1
  Data Type Conversion6/1 -> Gain10/1
  Data Type Conversion7/1 -> Gain12/1
  Data Type Conversion8/1 -> Gain13/1
  Data Type Conversion9/1 -> Gain14/1
  Data Type Conversion10/1 -> Gain4/1
  Data Type Conversion11/1 -> Gain5/1
  Data Type Conversion12/1 -> Gain9/1
  Data Type Conversion13/1 -> Gain11/1
  Data Type Conversion14/1 -> Gain15/1
  Gain7/1 -> Data Store Write2/1
  Gain1/1 -> Data Store Write5/1
  Gain2/1 -> Data Store Write/1
  Gain8/1 -> Data Store Write8/1
  Gain3/1 -> Data Store Write1/1
  Gain10/1 -> Data Store Write3/1
  Gain12/1 -> Data Store Write6/1
  Gain13/1 -> Data Store Write9/1
  Gain14/1 -> Data Store Write4/1
  Gain4/1 -> Data Store Write14/1
  Gain5/1 -> Data Store Write12/1
  Gain9/1 -> Data Store Write10/1
  Gain11/1 -> Data Store Write11/1
  Gain15/1 -> Data Store Write13/1
  Data Store Read/1 -> Bus Creator/1  "AI18"
  Data Store Read1/1 -> Bus Creator/2  "AI11"
  Data Store Read2/1 -> Bus Creator/3  "AI16"
  Data Store Read3/1 -> Bus Creator/4  "AI20"
  Data Store Read4/1 -> Bus Creator/5  "AI05"
  Data Store Read5/1 -> Bus Creator/6  "AI03"
  Data Store Read6/1 -> Bus Creator/7  "AI04"
  Data Store Read7/1 -> Bus Creator/8  "AI09"
  Data Store Read8/1 -> Bus Creator/9  "AI15"
  Data Store Read9/1 -> Bus Creator/10  "AI08"
  Data Store Read10/1 -> Bus Creator/11  "AI17"
  Data Store Read11/1 -> Bus Creator/12  "AI06"
  Data Store Read12/1 -> Bus Creator/13  "AI12"
  Data Store Read13/1 -> Bus Creator/14  "AI19"
  Data Store Read14/1 -> Bus Creator/15  "AI07"
  Bus Creator/1 -> AI/1

== system VehCtrl20260630_18B/SigIn/CAN0 ==
  ID : Inport
  Data : Inport  Port=2
  length : Inport  Port=3
  timestamp : Inport  Port=4
  function : TriggerPort  TriggerType=function-call  VariantControl=Variant
  AUTO1 : Subsystem
  AUTO2 : Subsystem
  AUTO3 : Subsystem
  Bus Creator : BusCreator  Inputs=2
  Bus Creator1 : BusCreator  Inputs=4
  Bus Creator2 : BusCreator  Inputs=3
  DC-DC_Msg : Subsystem
  PTC1 : Subsystem
  PTC2 : Subsystem
  RMT_VCU1 : Subsystem
  RMT_VCU2 : Subsystem
  RMT_VCU3 : Subsystem
  RMT_VCU4 : Subsystem
  PTC : Outport
  AUTO : Outport  Port=2
  DCDC : Outport  Port=3
  RMT : Outport  Port=4
  wires:
  length/1 -> [length]
  timestamp/1 -> [timestamp]
  Data/1 -> [Data]
  ID/1 -> [ID]
  [Data] -> PTC1/2(Data)
  [ID] -> PTC1/1(ID)
  [timestamp] -> PTC1/4(timestamp)
  [length] -> PTC1/3(length)
  [Data] -> PTC2/2(Data)
  PTC2/1(Message) -> Bus Creator/2
  [ID] -> PTC2/1(ID)
  [timestamp] -> PTC2/4(timestamp)
  [length] -> PTC2/3(length)
  Bus Creator/1 -> PTC/1
  PTC1/1(Message) -> Bus Creator/1
  AUTO2/1(Message) -> Bus Creator2/2
  [Data] -> AUTO2/2(Data)
  [ID] -> AUTO2/1(ID)
  Bus Creator2/1 -> AUTO/1
  AUTO1/1(Message) -> Bus Creator2/1
  [length] -> AUTO2/3(length)
  [ID] -> AUTO1/1(ID)
  [timestamp] -> AUTO1/4(timestamp)
  [Data] -> AUTO1/2(Data)
  [length] -> AUTO1/3(length)
  [timestamp] -> AUTO2/4(timestamp)
  [length] -> AUTO3/3(length)
  [Data] -> AUTO3/2(Data)
  [timestamp] -> AUTO3/4(timestamp)
  [ID] -> AUTO3/1(ID)
  AUTO3/1(Message) -> Bus Creator2/3
  DC-DC_Msg/1(Message) -> DCDC/1
  [length] -> DC-DC_Msg/3(length)
  [ID] -> DC-DC_Msg/1(ID)
  [Data] -> DC-DC_Msg/2(Data)
  [timestamp] -> DC-DC_Msg/4(timestamp)
  RMT_VCU4/1(Message) -> Bus Creator1/4  "RMT4"
  [ID] -> RMT_VCU3/1(ID)
  RMT_VCU2/1(Message) -> Bus Creator1/2  "RMT2"
  [length] -> RMT_VCU4/3(length)
  RMT_VCU3/1(Message) -> Bus Creator1/3  "RMT3"
  [Data] -> RMT_VCU2/2(Data)
  [ID] -> RMT_VCU4/1(ID)
  [Data] -> RMT_VCU1/2(Data)
  [timestamp] -> RMT_VCU1/4(timestamp)
  [ID] -> RMT_VCU1/1(ID)
  [timestamp] -> RMT_VCU3/4(timestamp)
  Bus Creator1/1 -> RMT/1
  RMT_VCU1/1(Message) -> Bus Creator1/1  "RMT1"
  [timestamp] -> RMT_VCU4/4(timestamp)
  [length] -> RMT_VCU2/3(length)
  [Data] -> RMT_VCU4/2(Data)
  [length] -> RMT_VCU1/3(length)
  [length] -> RMT_VCU3/3(length)
  [Data] -> RMT_VCU3/2(Data)
  [timestamp] -> RMT_VCU2/4(timestamp)
  [ID] -> RMT_VCU2/1(ID)
